simulink model "mrefrobotarm_previous_y_previous_u_previous_ref_cover_test_2"  (R2018b)
settings: Solver=FixedStepAuto  StartTime=0.0  StopTime=20  RelTol=1e-3  AbsTol=1e-6
undefined symbols (not defined in the file or in its folder): cc, options
libraries: neural x132, simulink x2
(part 4 of 6)

== system mrefrobotarm_previous_y_previous_u_previous_ref_cover_test_2/Feed-Forward Neural Network/Layer 3/Delays 1 ==
  "p{3}" : Inport  PortDimensions=30
      mask Display: e = 0.06;c1 = [120 230 180]/255;c2 = ([120 230 180]+0)/(256+128);c3 = ([120 230 180]+128)/(256+128);patch([0 1 1 0],[0 0 1 1],c1);patch([0 1 1 1-e 1-e 0+e],[0 0 1 1-e 0+e 0+e],c2);patch([0 0 1 1-e 0+e 0+e],[0 1 1 1-e 1-e 0+e],c3);plot([0 1 1 0 0],[0 0 1 1 0]);
  mux : Mux  Inputs=1
      mask Display: e = 0.06;c1 = [120 150 230]/255;c2 = ([120 150 230]+0)/383;c3 = ([120 150 230]+128)/383;patch([0 1 1 0],[0 0 1 1],c1);patch([0 1 1 1-e 1-e 0+e],[0 0 1 1-e 0+e 0+e],c2);patch([0 0 1 1-e 0+e 0+e],[0 1 1 1-e 1-e 0+e],c3);plot([0 1 1 0 0],[0 0 1 1 0]);disp('Mux')
  "pd{3,2}" : Outport
      mask Display: e = 0.06;c1 = [120 230 180]/255;c2 = ([120 230 180]+0)/(256+128);c3 = ([120 230 180]+128)/(256+128);patch([0 1 1 0],[0 0 1 1],c1);patch([0 1 1 1-e 1-e 0+e],[0 0 1 1-e 0+e 0+e],c2);patch([0 0 1 1-e 0+e 0+e],[0 1 1 1-e 1-e 0+e],c3);plot([0 1 1 0 0],[0 0 1 1 0]);
  wires:
  "p{3}"/1 -> mux/1
  mux/1 -> "pd{3,2}"/1

== system mrefrobotarm_previous_y_previous_u_previous_ref_cover_test_2/Feed-Forward Neural Network/Layer 3/LW{3,2} ==
  "ad{3,2}" : Inport  PortDimensions=30
      mask Display: e = 0.06;c1 = [120 230 180]/255;c2 = ([120 230 180]+0)/(256+128);c3 = ([120 230 180]+128)/(256+128);patch([0 1 1 0],[0 0 1 1],c1);patch([0 1 1 1-e 1-e 0+e],[0 0 1 1-e 0+e 0+e],c2);patch([0 0 1 1-e 0+e 0+e],[0 1 1 1-e 1-e 0+e],c3);plot([0 1 1 0 0],[0 0 1 1 0]);
  "IW{3,2}(1,:)'" : Constant  Value=[-0.179633159964680266806880126750911585986614227294921875;-0.01072873765062364037614628387018456123769283294677734375;-0.0291453057248748058360998669513719505630433559417724609375;0.05859045612955075810202032471352140419185161590576171875;-0.237638764700321913903025006220559589564800262451171875;-0.209838527725091539277713081901310943067073822021484375;-0.27791655307496510030063063823035918176174163818359375;-0.07008976059233355815347721318175899796187877655029296875;-0.11554327471293225626514100667918683029711246490478515625;0.27212249906517038677833397741778753697872161865234375;-0.1734031338030869451305449047140427865087985992431640625;0.0536763624525791460673218580268439836800098419189453125;-0.037173437880853761605681739865758572705090045928955078125;0.1358518131119930971717479906146763823926448822021484375;-0.11157815841815578450368917629020870663225650787353515625;-0.023913464068717076027592582931902143172919750213623046875;-0.4313994517536372530486232790281064808368682861328125;0.1636875861604869808463291747102630324661731719970703125;0.037232113811342650022684352961732656694948673248291015625;-0.52644415726454052428806562602403573691844940185546875;0.039897217969779720514456045066253864206373691558837890625;-0.1369287872106144388073545314910006709396839141845703125;0.44593864887069745162051503939437679946422576904296875;0.410742338437982856813590615274733863770961761474609375;-0.145121658875231818175421949490555562078952789306640625;0.06655502995710448066457587401600903831422328948974609375;-0.418109406113754300537976860141498036682605743408203125;0.11096998879556761730125202802810235880315303802490234375;0.333827163986122277261614499366260133683681488037109375;0.186101897373585012385177606120123527944087982177734375]
      mask Display: e = 0.06;c1 = [120 150 230]/255;c2 = ([120 150 230]+0)/383;c3 = ([120 150 230]+128)/383;patch([0 1 1 0],[0 0 1 1],c1);patch([0 1 1 1-e 1-e 0+e],[0 0 1 1-e 0+e 0+e],c2);patch([0 0 1 1-e 0+e 0+e],[0 1 1 1-e 1-e 0+e],c3);plot([0 1 1 0 0],[0 0 1 1 0]);disp('weights');
  Mux : Mux  Inputs=1
      mask Display: e = 0.06;c1 = [120 150 230]/255;c2 = ([120 150 230]+0)/383;c3 = ([120 150 230]+128)/383;patch([0 1 1 0],[0 0 1 1],c1);patch([0 1 1 1-e 1-e 0+e],[0 0 1 1-e 0+e 0+e],c2);patch([0 0 1 1-e 0+e 0+e],[0 1 1 1-e 1-e 0+e],c3);plot([0 1 1 0 0],[0 0 1 1 0]);disp('Mux');
  dotprod1 : neural/Weight Functions/dotprod
  "lz{3,2}" : Outport
      mask Display: e = 0.06;c1 = [120 230 180]/255;c2 = ([120 230 180]+0)/(256+128);c3 = ([120 230 180]+128)/(256+128);patch([0 1 1 0],[0 0 1 1],c1);patch([0 1 1 1-e 1-e 0+e],[0 0 1 1-e 0+e 0+e],c2);patch([0 0 1 1-e 0+e 0+e],[0 1 1 1-e 1-e 0+e],c3);plot([0 1 1 0 0],[0 0 1 1 0]);
  wires:
  "IW{3,2}(1,:)'"/1 -> dotprod1/1
  "ad{3,2}"/1 -> dotprod1/2
  dotprod1/1 -> Mux/1
  Mux/1 -> "lz{3,2}"/1

== system mrefrobotarm_previous_y_previous_u_previous_ref_cover_test_2/Feed-Forward Neural Network1/Layer 1/Delays 1 ==
  "p{1}" : Inport  PortDimensions=10
      mask Display: e = 0.06;c1 = [120 230 180]/255;c2 = ([120 230 180]+0)/(256+128);c3 = ([120 230 180]+128)/(256+128);patch([0 1 1 0],[0 0 1 1],c1);patch([0 1 1 1-e 1-e 0+e],[0 0 1 1-e 0+e 0+e],c2);patch([0 0 1 1-e 0+e 0+e],[0 1 1 1-e 1-e 0+e],c3);plot([0 1 1 0 0],[0 0 1 1 0]);
  mux : Mux  Inputs=1
      mask Display: e = 0.06;c1 = [120 150 230]/255;c2 = ([120 150 230]+0)/383;c3 = ([120 150 230]+128)/383;patch([0 1 1 0],[0 0 1 1],c1);patch([0 1 1 1-e 1-e 0+e],[0 0 1 1-e 0+e 0+e],c2);patch([0 0 1 1-e 0+e 0+e],[0 1 1 1-e 1-e 0+e],c3);plot([0 1 1 0 0],[0 0 1 1 0]);disp('Mux')
  "pd{1,1}" : Outport
      mask Display: e = 0.06;c1 = [120 230 180]/255;c2 = ([120 230 180]+0)/(256+128);c3 = ([120 230 180]+128)/(256+128);patch([0 1 1 0],[0 0 1 1],c1);patch([0 1 1 1-e 1-e 0+e],[0 0 1 1-e 0+e 0+e],c2);patch([0 0 1 1-e 0+e 0+e],[0 1 1 1-e 1-e 0+e],c3);plot([0 1 1 0 0],[0 0 1 1 0]);
  wires:
  "p{1}"/1 -> mux/1
  mux/1 -> "pd{1,1}"/1

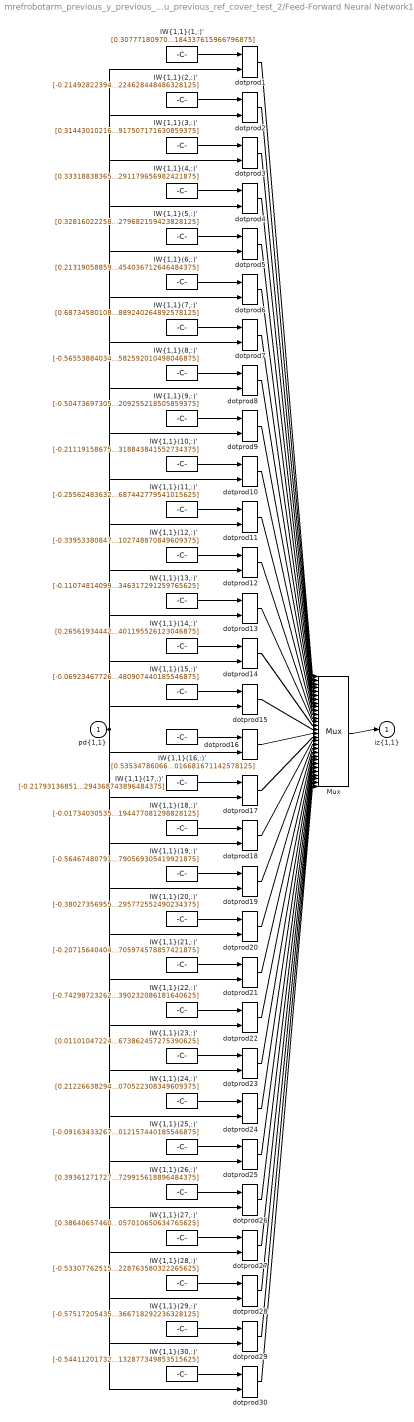
== system mrefrobotarm_previous_y_previous_u_previous_ref_cover_test_2/Feed-Forward Neural Network1/Layer 1/IW{1,1} ==
  "pd{1,1}" : Inport  PortDimensions=10
      mask Display: e = 0.06;c1 = [120 230 180]/255;c2 = ([120 230 180]+0)/(256+128);c3 = ([120 230 180]+128)/(256+128);patch([0 1 1 0],[0 0 1 1],c1);patch([0 1 1 1-e 1-e 0+e],[0 0 1 1-e 0+e 0+e],c2);patch([0 0 1 1-e 0+e 0+e],[0 1 1 1-e 1-e 0+e],c3);plot([0 1 1 0 0],[0 0 1 1 0]);
  "IW{1,1}(1,:)'" : Constant  Value=[0.307771809704280141506416157426428981125354766845703125;-0.043494246471554913469059755470880190841853618621826171875;-0.038310852488129772119851423894942854531109333038330078125;-0.39541211499447570520970884899725206196308135986328125;-0.70069751174348116062873259579646401107311248779296875;0.65787882665114827407393249814049340784549713134765625;-0.444848337035453955667918535255012102425098419189453125;-0.534193590442934240769545795046724379062652587890625;-0.452507108681440561870346073192195035517215728759765625;0.5736423354881441394326202498632483184337615966796875]
      mask Display: e = 0.06;c1 = [120 150 230]/255;c2 = ([120 150 230]+0)/383;c3 = ([120 150 230]+128)/383;patch([0 1 1 0],[0 0 1 1],c1);patch([0 1 1 1-e 1-e 0+e],[0 0 1 1-e 0+e 0+e],c2);patch([0 0 1 1-e 0+e 0+e],[0 1 1 1-e 1-e 0+e],c3);plot([0 1 1 0 0],[0 0 1 1 0]);disp('Weights');
  "IW{1,1}(10,:)'" : Constant  Value=[-0.2111915867591773465772320150790619663894176483154296875;-0.42392787982224933163166724625625647604465484619140625;0.313182134356018437859603409378905780613422393798828125;0.8660538287659613754243537186994217336177825927734375;0.465944929849588296288942501632845960557460784912109375;-0.317882144322859605534148386141168884932994842529296875;0.5471005603664356176096816852805204689502716064453125;0.048378896684587037457792035866077640093863010406494140625;0.88527457170474466163767601756262592971324920654296875;-0.06293203749796126567073173418975784443318843841552734375]
      mask Display: e = 0.06;c1 = [120 150 230]/255;c2 = ([120 150 230]+0)/383;c3 = ([120 150 230]+128)/383;patch([0 1 1 0],[0 0 1 1],c1);patch([0 1 1 1-e 1-e 0+e],[0 0 1 1-e 0+e 0+e],c2);patch([0 0 1 1-e 0+e 0+e],[0 1 1 1-e 1-e 0+e],c3);plot([0 1 1 0 0],[0 0 1 1 0]);disp('Weights');
  "IW{1,1}(11,:)'" : Constant  Value=[-0.255624836328040394572980176235432736575603485107421875;0.44469153543896167146698417127481661736965179443359375;0.58810225130934201676069505992927588522434234619140625;-0.381773211793491717980231214824016205966472625732421875;0.636150888388204549528381903655827045440673828125;-0.160165825236976699930124823367805220186710357666015625;0.361341451607977981463903915937407873570919036865234375;0.428811830416127082177268903251388110220432281494140625;-0.372886982074612571835814378573559224605560302734375;0.401883345447998918675835966496379114687442779541015625]
      mask Display: e = 0.06;c1 = [120 150 230]/255;c2 = ([120 150 230]+0)/383;c3 = ([120 150 230]+128)/383;patch([0 1 1 0],[0 0 1 1],c1);patch([0 1 1 1-e 1-e 0+e],[0 0 1 1-e 0+e 0+e],c2);patch([0 0 1 1-e 0+e 0+e],[0 1 1 1-e 1-e 0+e],c3);plot([0 1 1 0 0],[0 0 1 1 0]);disp('Weights');
  "IW{1,1}(12,:)'" : Constant  Value=[-0.339533808477128939973255228323978371918201446533203125;0.539710960120284966023973538540303707122802734375;-0.7230875453157439292084518456249497830867767333984375;-0.75990866812186597112344088600366376340389251708984375;-0.354088287837987625294999816105701029300689697265625;-0.353970240989271711651298346623661927878856658935546875;-0.10842578628777639615510253179309074766933917999267578125;-0.01447441056256725845641231131821768940426409244537353515625;-0.456615513925438809561541120274341665208339691162109375;-0.261220551168401760033788150394684635102748870849609375]
      mask Display: e = 0.06;c1 = [120 150 230]/255;c2 = ([120 150 230]+0)/383;c3 = ([120 150 230]+128)/383;patch([0 1 1 0],[0 0 1 1],c1);patch([0 1 1 1-e 1-e 0+e],[0 0 1 1-e 0+e 0+e],c2);patch([0 0 1 1-e 0+e 0+e],[0 1 1 1-e 1-e 0+e],c3);plot([0 1 1 0 0],[0 0 1 1 0]);disp('Weights');
  "IW{1,1}(13,:)'" : Constant  Value=[-0.110748140990551302564881552825681865215301513671875;0.66488624107314231448384589384659193456172943115234375;-1.00451912367756523991602080059237778186798095703125;-0.0143360503455160250008137978738886886276304721832275390625;0.6747034829726137328265167525387369096279144287109375;0.037869992030076689293327518726073321886360645294189453125;-0.2233703071642894055770511840819381177425384521484375;0.1543495324337380847357081847803783603012561798095703125;-0.6817280066758144574379230107297189533710479736328125;-0.25424477166286740814626909923390485346317291259765625]
      mask Display: e = 0.06;c1 = [120 150 230]/255;c2 = ([120 150 230]+0)/383;c3 = ([120 150 230]+128)/383;patch([0 1 1 0],[0 0 1 1],c1);patch([0 1 1 1-e 1-e 0+e],[0 0 1 1-e 0+e 0+e],c2);patch([0 0 1 1-e 0+e 0+e],[0 1 1 1-e 1-e 0+e],c3);plot([0 1 1 0 0],[0 0 1 1 0]);disp('Weights');
  "IW{1,1}(14,:)'" : Constant  Value=[0.265619344429818438069190733585855923593044281005859375;-0.282970550854229341286583121473086066544055938720703125;-0.5838578775873510817717715326580218970775604248046875;0.294580978398594428568912917398847639560699462890625;0.64224270360970781013065789011307060718536376953125;-0.17698999119896263731988028666819445788860321044921875;-0.06350503851383948461517547912080772221088409423828125;0.58935462278309425077083005817257799208164215087890625;0.62621659979370136728249462976236827671527862548828125;0.1318430666219640723380024383004638366401195526123046875]
      mask Display: e = 0.06;c1 = [120 150 230]/255;c2 = ([120 150 230]+0)/383;c3 = ([120 150 230]+128)/383;patch([0 1 1 0],[0 0 1 1],c1);patch([0 1 1 1-e 1-e 0+e],[0 0 1 1-e 0+e 0+e],c2);patch([0 0 1 1-e 0+e 0+e],[0 1 1 1-e 1-e 0+e],c3);plot([0 1 1 0 0],[0 0 1 1 0]);disp('Weights');
  "IW{1,1}(15,:)'" : Constant  Value=[-0.069234677267842936743136306176893413066864013671875;0.357620645651575530532539914929657243192195892333984375;0.024739682030093586295738106173303094692528247833251953125;0.406580565759079914922580201164237223565578460693359375;-0.1414763552845024197068823923473246395587921142578125;0.77379347285040334103456416414701379835605621337890625;0.54400482337093336582256597466766834259033203125;0.257672646340499966743919912914861924946308135986328125;0.4042055275314468953951063667773269116878509521484375;0.6191001141682999087123562276246957480907440185546875]
      mask Display: e = 0.06;c1 = [120 150 230]/255;c2 = ([120 150 230]+0)/383;c3 = ([120 150 230]+128)/383;patch([0 1 1 0],[0 0 1 1],c1);patch([0 1 1 1-e 1-e 0+e],[0 0 1 1-e 0+e 0+e],c2);patch([0 0 1 1-e 0+e 0+e],[0 1 1 1-e 1-e 0+e],c3);plot([0 1 1 0 0],[0 0 1 1 0]);disp('Weights');
  "IW{1,1}(16,:)'" : Constant  Value=[0.5353478606635488912246501058689318597316741943359375;-0.298798871045879599339656351730809547007083892822265625;-0.306842919989221252219380176029517315328121185302734375;0.79214491503970763108810615449328906834125518798828125;0.107274974298643910319839278599829412996768951416015625;-0.04982289745277827808234150097632664255797863006591796875;0.1398078294476846339389197737546055577695369720458984375;0.73950277251963658642353038885630667209625244140625;0.0214329040625382515050656451194299734197556972503662109375;-0.59363821103110503418776033868198283016681671142578125]
      mask Display: e = 0.06;c1 = [120 150 230]/255;c2 = ([120 150 230]+0)/383;c3 = ([120 150 230]+128)/383;patch([0 1 1 0],[0 0 1 1],c1);patch([0 1 1 1-e 1-e 0+e],[0 0 1 1-e 0+e 0+e],c2);patch([0 0 1 1-e 0+e 0+e],[0 1 1 1-e 1-e 0+e],c3);plot([0 1 1 0 0],[0 0 1 1 0]);disp('Weights');
  "IW{1,1}(17,:)'" : Constant  Value=[-0.2179313685150011392632762863286188803613185882568359375;0.02389454008851725486106687412757310084998607635498046875;0.80226571345702046844650112689123488962650299072265625;0.33127862043797751123719308452564291656017303466796875;-0.47181821059433415310735426828614436089992523193359375;0.0302617469843945753604774751011063926853239536285400390625;0.78373483792398135339141163058229722082614898681640625;-0.033101967548309345346080334593352745287120342254638671875;-0.06509617185323690602416490946779958903789520263671875;-0.4540540617562258685069309649406932294368743896484375]
      mask Display: e = 0.06;c1 = [120 150 230]/255;c2 = ([120 150 230]+0)/383;c3 = ([120 150 230]+128)/383;patch([0 1 1 0],[0 0 1 1],c1);patch([0 1 1 1-e 1-e 0+e],[0 0 1 1-e 0+e 0+e],c2);patch([0 0 1 1-e 0+e 0+e],[0 1 1 1-e 1-e 0+e],c3);plot([0 1 1 0 0],[0 0 1 1 0]);disp('Weights');
  "IW{1,1}(18,:)'" : Constant  Value=[-0.017340305353522177111980084873721352778375148773193359375;0.04635262968849508669055836662664660252630710601806640625;0.49087893166783247433926362646161578595638275146484375;0.261355444844639184243106910798815079033374786376953125;0.038895872356487219689835654889975558035075664520263671875;0.76061985589617275849150246358476579189300537109375;0.16038243618602454620969410825637169182300567626953125;0.269770227677864460336110141724930144846439361572265625;0.85486484585484101561547731762402690947055816650390625;-0.474622970419836420763459727822919376194477081298828125]
      mask Display: e = 0.06;c1 = [120 150 230]/255;c2 = ([120 150 230]+0)/383;c3 = ([120 150 230]+128)/383;patch([0 1 1 0],[0 0 1 1],c1);patch([0 1 1 1-e 1-e 0+e],[0 0 1 1-e 0+e 0+e],c2);patch([0 0 1 1-e 0+e 0+e],[0 1 1 1-e 1-e 0+e],c3);plot([0 1 1 0 0],[0 0 1 1 0]);disp('Weights');
  "IW{1,1}(19,:)'" : Constant  Value=[-0.56467480791342705703783622084301896393299102783203125;-0.0030660566154840085406618754859664477407932281494140625;-0.342498503655595476491413364783511497080326080322265625;-0.22528161666232360271777679372462444007396697998046875;0.06229949556277590561048640438457368873059749603271484375;-0.856195965195246433410147801623679697513580322265625;0.56695735295288007815628361640847288072109222412109375;-0.18273876771567143517671638619503937661647796630859375;-0.39019604298290000432558599641197361052036285400390625;-0.643270272670612097698494835640303790569305419921875]
      mask Display: e = 0.06;c1 = [120 150 230]/255;c2 = ([120 150 230]+0)/383;c3 = ([120 150 230]+128)/383;patch([0 1 1 0],[0 0 1 1],c1);patch([0 1 1 1-e 1-e 0+e],[0 0 1 1-e 0+e 0+e],c2);patch([0 0 1 1-e 0+e 0+e],[0 1 1 1-e 1-e 0+e],c3);plot([0 1 1 0 0],[0 0 1 1 0]);disp('Weights');
  "IW{1,1}(2,:)'" : Constant  Value=[-0.2149282239453440268572848026451538316905498504638671875;0.50939800546889235643988058654940687119960784912109375;-0.570595278838305741686554029001854360103607177734375;-0.6491838212484617454123281277134083211421966552734375;0.524588753903739490880298035335727035999298095703125;-0.325806575234383277717142846086062490940093994140625;0.4073454672740408621933738686493597924709320068359375;0.1445179480051441978094572959889774210751056671142578125;0.557599898389703252377103126491419970989227294921875;-0.33629203092728687796153508315910585224628448486328125]
      mask Display: e = 0.06;c1 = [120 150 230]/255;c2 = ([120 150 230]+0)/383;c3 = ([120 150 230]+128)/383;patch([0 1 1 0],[0 0 1 1],c1);patch([0 1 1 1-e 1-e 0+e],[0 0 1 1-e 0+e 0+e],c2);patch([0 0 1 1-e 0+e 0+e],[0 1 1 1-e 1-e 0+e],c3);plot([0 1 1 0 0],[0 0 1 1 0]);disp('Weights');
  "IW{1,1}(20,:)'" : Constant  Value=[-0.380273569552752876976597917746403254568576812744140625;-0.430511165009204999076786180012277327477931976318359375;0.354253288781558206554933576626353897154331207275390625;0.445619148653988272901216305399429984390735626220703125;-0.60980214170925106653697866931906901299953460693359375;0.60264849482189231100193183010560460388660430908203125;0.286226129170386867084374671321711502969264984130859375;0.296664076206746951669401823892258107662200927734375;-0.38376606122486578431818315948476083576679229736328125;0.1592426923493431567546707583460374735295772552490234375]
      mask Display: e = 0.06;c1 = [120 150 230]/255;c2 = ([120 150 230]+0)/383;c3 = ([120 150 230]+128)/383;patch([0 1 1 0],[0 0 1 1],c1);patch([0 1 1 1-e 1-e 0+e],[0 0 1 1-e 0+e 0+e],c2);patch([0 0 1 1-e 0+e 0+e],[0 1 1 1-e 1-e 0+e],c3);plot([0 1 1 0 0],[0 0 1 1 0]);disp('Weights');
  "IW{1,1}(21,:)'" : Constant  Value=[-0.20715640404519952699757823211257345974445343017578125;0.9811699028163343161423881610971875488758087158203125;-0.001095329187504811944975369186749958316795527935028076171875;-0.277444713932339770412482948813703842461109161376953125;0.55580805253002185661870271360385231673717498779296875;-0.64553407503771043085549763418384827673435211181640625;-0.422001384311685712180661766979028470814228057861328125;0.393923183878474636454569690613425336778163909912109375;0.083918194813454027869425999597297050058841705322265625;-0.283713183453508654974228875289554707705974578857421875]
      mask Display: e = 0.06;c1 = [120 150 230]/255;c2 = ([120 150 230]+0)/383;c3 = ([120 150 230]+128)/383;patch([0 1 1 0],[0 0 1 1],c1);patch([0 1 1 1-e 1-e 0+e],[0 0 1 1-e 0+e 0+e],c2);patch([0 0 1 1-e 0+e 0+e],[0 1 1 1-e 1-e 0+e],c3);plot([0 1 1 0 0],[0 0 1 1 0]);disp('Weights');
  "IW{1,1}(22,:)'" : Constant  Value=[-0.74298723262986421378428758544032461941242218017578125;-0.474285430413762976176172969644539989531040191650390625;-0.2219220129482323555780709511964232660830020904541015625;-0.07774456600170388809178945166422636248171329498291015625;0.159011878942632634004183955767075531184673309326171875;-0.474236493815869242229865676563349552452564239501953125;-0.34955980920388896038275561295449733734130859375;0.263576614616158944048862622366868890821933746337890625;0.656227952555379356880393970641307532787322998046875;0.495996797371051345582060321248718537390232086181640625]
      mask Display: e = 0.06;c1 = [120 150 230]/255;c2 = ([120 150 230]+0)/383;c3 = ([120 150 230]+128)/383;patch([0 1 1 0],[0 0 1 1],c1);patch([0 1 1 1-e 1-e 0+e],[0 0 1 1-e 0+e 0+e],c2);patch([0 0 1 1-e 0+e 0+e],[0 1 1 1-e 1-e 0+e],c3);plot([0 1 1 0 0],[0 0 1 1 0]);disp('Weights');
  "IW{1,1}(23,:)'" : Constant  Value=[0.01101047224694271138567547296815973822958767414093017578125;-0.83652318268884062746337804128415882587432861328125;-0.6720858263646014574277387509937398135662078857421875;0.06519613312673551430709295573251438327133655548095703125;-0.288183944151695625723874627510667778551578521728515625;-0.48909683596764808033441340739955194294452667236328125;0.54268768030462333218366666187648661434650421142578125;-0.0153055303761240289739387065992559655569493770599365234375;0.1757264020219303224390472450977540574967861175537109375;-0.293937485561877986928180916947894729673862457275390625]
      mask Display: e = 0.06;c1 = [120 150 230]/255;c2 = ([120 150 230]+0)/383;c3 = ([120 150 230]+128)/383;patch([0 1 1 0],[0 0 1 1],c1);patch([0 1 1 1-e 1-e 0+e],[0 0 1 1-e 0+e 0+e],c2);patch([0 0 1 1-e 0+e 0+e],[0 1 1 1-e 1-e 0+e],c3);plot([0 1 1 0 0],[0 0 1 1 0]);disp('Weights');
  "IW{1,1}(24,:)'" : Constant  Value=[0.2122663829425259496286315652469056658446788787841796875;0.87923061827891757502584368921816349029541015625;-0.5173249006417501849597329055541194975376129150390625;-0.50307150349048967985510216749389655888080596923828125;0.1947665745272291193401770215132273733615875244140625;0.26726591958569378970622665292466990649700164794921875;-0.128537570280304602743370878670248202979564666748046875;-0.4015021175823199062193680219934321939945220947265625;0.71182418664467472790846613861504010856151580810546875;-0.122855789206089749399097854620777070522308349609375]
      mask Display: e = 0.06;c1 = [120 150 230]/255;c2 = ([120 150 230]+0)/383;c3 = ([120 150 230]+128)/383;patch([0 1 1 0],[0 0 1 1],c1);patch([0 1 1 1-e 1-e 0+e],[0 0 1 1-e 0+e 0+e],c2);patch([0 0 1 1-e 0+e 0+e],[0 1 1 1-e 1-e 0+e],c3);plot([0 1 1 0 0],[0 0 1 1 0]);disp('Weights');
  "IW{1,1}(25,:)'" : Constant  Value=[-0.09163433267084818145686853085862821899354457855224609375;-0.79242044992990423590839554890408180654048919677734375;-0.100048388071002858357161358071607537567615509033203125;0.1508863568801963317422831778458203189074993133544921875;-0.52491946330139238607870311170700006186962127685546875;-0.9073207461986847466306471687857992947101593017578125;0.305921576666395356181027409547823481261730194091796875;-0.28550897310796197192672707387828268110752105712890625;0.3700650003189187575713958722190000116825103759765625;0.01483537959348367289702519400407254579477012157440185546875]
      mask Display: e = 0.06;c1 = [120 150 230]/255;c2 = ([120 150 230]+0)/383;c3 = ([120 150 230]+128)/383;patch([0 1 1 0],[0 0 1 1],c1);patch([0 1 1 1-e 1-e 0+e],[0 0 1 1-e 0+e 0+e],c2);patch([0 0 1 1-e 0+e 0+e],[0 1 1 1-e 1-e 0+e],c3);plot([0 1 1 0 0],[0 0 1 1 0]);disp('Weights');
  "IW{1,1}(26,:)'" : Constant  Value=[0.393612717278230495043800374332931824028491973876953125;0.2449765807941226558597236362402327358722686767578125;-0.03009018765526084993044975135489949025213718414306640625;0.14629061622603833914268989246920682489871978759765625;0.439887108136198412555728509687469340860843658447265625;0.435562173454939915995254295921768061816692352294921875;0.336788968183238723863581753903417848050594329833984375;-0.428207393410589443050184854655526578426361083984375;-0.054417900950539950521989140952427987940609455108642578125;1.0199853001420409182031789896427653729915618896484375]
      mask Display: e = 0.06;c1 = [120 150 230]/255;c2 = ([120 150 230]+0)/383;c3 = ([120 150 230]+128)/383;patch([0 1 1 0],[0 0 1 1],c1);patch([0 1 1 1-e 1-e 0+e],[0 0 1 1-e 0+e 0+e],c2);patch([0 0 1 1-e 0+e 0+e],[0 1 1 1-e 1-e 0+e],c3);plot([0 1 1 0 0],[0 0 1 1 0]);disp('Weights');
  "IW{1,1}(27,:)'" : Constant  Value=[0.386406574607860431314065863261930644512176513671875;0.469835350060989143106127130522509105503559112548828125;-0.3691521633424239556831025765859521925449371337890625;-0.45968636278126029370838523391284979879856109619140625;-0.12253896032814211303207940773063455708324909210205078125;0.51055111602274383386657063965685665607452392578125;-0.25427556952147067903524657594971358776092529296875;0.4000694399878466089859330168110318481922149658203125;0.5497090132858077904387528178631328046321868896484375;0.62451276436301006445006578360334970057010650634765625]
      mask Display: e = 0.06;c1 = [120 150 230]/255;c2 = ([120 150 230]+0)/383;c3 = ([120 150 230]+128)/383;patch([0 1 1 0],[0 0 1 1],c1);patch([0 1 1 1-e 1-e 0+e],[0 0 1 1-e 0+e 0+e],c2);patch([0 0 1 1-e 0+e 0+e],[0 1 1 1-e 1-e 0+e],c3);plot([0 1 1 0 0],[0 0 1 1 0]);disp('Weights');
  "IW{1,1}(28,:)'" : Constant  Value=[-0.5330776251530677800616331296623684465885162353515625;-0.09896275413630002681930619701233808882534503936767578125;0.59870269426114497424151750237797386944293975830078125;0.6583543298551373101901162954163737595081329345703125;0.62137262912390955893471300441888161003589630126953125;0.0274271679633210745119509255118828150443732738494873046875;-0.386383313608881895362401337479241192340850830078125;-0.373521518345400205252104797182255424559116363525390625;-0.1745289113787924784038096959193353541195392608642578125;-0.68166057721812711722719768658862449228763580322265625]
      mask Display: e = 0.06;c1 = [120 150 230]/255;c2 = ([120 150 230]+0)/383;c3 = ([120 150 230]+128)/383;patch([0 1 1 0],[0 0 1 1],c1);patch([0 1 1 1-e 1-e 0+e],[0 0 1 1-e 0+e 0+e],c2);patch([0 0 1 1-e 0+e 0+e],[0 1 1 1-e 1-e 0+e],c3);plot([0 1 1 0 0],[0 0 1 1 0]);disp('Weights');
  "IW{1,1}(29,:)'" : Constant  Value=[-0.57517205435042340067042232476524077355861663818359375;0.63308192763810922087941435165703296661376953125;-0.09556525966967858998213358745488221757113933563232421875;-0.5584199775632636697508814904722385108470916748046875;0.345765858847536577957981762665440328419208526611328125;0.08596895869872944739853437567944638431072235107421875;-0.1846575835968873591230732245094259269535541534423828125;0.65145079957593632347112588831805624067783355712890625;-0.501689780634055892960532219149172306060791015625;-0.61266191132330505286773814077605493366718292236328125]
      mask Display: e = 0.06;c1 = [120 150 230]/255;c2 = ([120 150 230]+0)/383;c3 = ([120 150 230]+128)/383;patch([0 1 1 0],[0 0 1 1],c1);patch([0 1 1 1-e 1-e 0+e],[0 0 1 1-e 0+e 0+e],c2);patch([0 0 1 1-e 0+e 0+e],[0 1 1 1-e 1-e 0+e],c3);plot([0 1 1 0 0],[0 0 1 1 0]);disp('Weights');
  "IW{1,1}(3,:)'" : Constant  Value=[0.314430102162298330537026913589215837419033050537109375;0.276695513253253644325724280861322768032550811767578125;0.11751958538400335274598518253696965985000133514404296875;0.1846764705887174173870590720980544574558734893798828125;-0.64765345192008594299437618246884085237979888916015625;-0.69717973432415181189725217336672358214855194091796875;0.1215129375684755042019702386824064888060092926025390625;0.38445320860246934291382103765499778091907501220703125;0.74698130652669891826889170260983519256114959716796875;0.297597636979915092236836926531395874917507171630859375]
      mask Display: e = 0.06;c1 = [120 150 230]/255;c2 = ([120 150 230]+0)/383;c3 = ([120 150 230]+128)/383;patch([0 1 1 0],[0 0 1 1],c1);patch([0 1 1 1-e 1-e 0+e],[0 0 1 1-e 0+e 0+e],c2);patch([0 0 1 1-e 0+e 0+e],[0 1 1 1-e 1-e 0+e],c3);plot([0 1 1 0 0],[0 0 1 1 0]);disp('Weights');
  "IW{1,1}(30,:)'" : Constant  Value=[-0.54411201732523573060262833678280003368854522705078125;-0.1570049627788529245098203546149306930601596832275390625;0.4750648553590675060576131727430038154125213623046875;-0.332924171479602348799886613051057793200016021728515625;0.336816257924666573320138240887899883091449737548828125;0.0772141881037635702256238801055587828159332275390625;0.138879371464563750038223588489927351474761962890625;-0.7413902499064313200705100825871340930461883544921875;-0.556925916111620011861305101774632930755615234375;-0.379493537000827940719460684704245068132877349853515625]
      mask Display: e = 0.06;c1 = [120 150 230]/255;c2 = ([120 150 230]+0)/383;c3 = ([120 150 230]+128)/383;patch([0 1 1 0],[0 0 1 1],c1);patch([0 1 1 1-e 1-e 0+e],[0 0 1 1-e 0+e 0+e],c2);patch([0 0 1 1-e 0+e 0+e],[0 1 1 1-e 1-e 0+e],c3);plot([0 1 1 0 0],[0 0 1 1 0]);disp('Weights');
  "IW{1,1}(4,:)'" : Constant  Value=[0.333188383657982922780860235434374772012233734130859375;-0.8119891062851021246160598821006715297698974609375;-0.43539581511156633109038693874026648700237274169921875;0.115329974937103341137145662287366576492786407470703125;-0.410897767185643358889279852519393898546695709228515625;-0.1653380888177397867178086698913830332458019256591796875;-0.66921948665613950613106908349436707794666290283203125;0.2423332585656756965608593645811197347939014434814453125;0.352153723637267657142757570909452624619007110595703125;-0.471892129319398001552343657749588601291179656982421875]
      mask Display: e = 0.06;c1 = [120 150 230]/255;c2 = ([120 150 230]+0)/383;c3 = ([120 150 230]+128)/383;patch([0 1 1 0],[0 0 1 1],c1);patch([0 1 1 1-e 1-e 0+e],[0 0 1 1-e 0+e 0+e],c2);patch([0 0 1 1-e 0+e 0+e],[0 1 1 1-e 1-e 0+e],c3);plot([0 1 1 0 0],[0 0 1 1 0]);disp('Weights');
  "IW{1,1}(5,:)'" : Constant  Value=[0.328160222582545901826023282410460524260997772216796875;0.11696869091104332427644152403445332311093807220458984375;-0.56572687517270459078844169198418967425823211669921875;-0.044997049681217267391719616398404468782246112823486328125;-0.414037671684482855294362479980918578803539276123046875;-0.6718978551824748013387988976319320499897003173828125;0.11602708978398555694777627422809018753468990325927734375;-0.28088853726513984820911673523369245231151580810546875;-0.1101044169173044096066149677426437847316265106201171875;0.72922980289897498806794828851707279682159423828125]
      mask Display: e = 0.06;c1 = [120 150 230]/255;c2 = ([120 150 230]+0)/383;c3 = ([120 150 230]+128)/383;patch([0 1 1 0],[0 0 1 1],c1);patch([0 1 1 1-e 1-e 0+e],[0 0 1 1-e 0+e 0+e],c2);patch([0 0 1 1-e 0+e 0+e],[0 1 1 1-e 1-e 0+e],c3);plot([0 1 1 0 0],[0 0 1 1 0]);disp('Weights');
  "IW{1,1}(6,:)'" : Constant  Value=[0.2131905885959748669922220187800121493637561798095703125;-0.5860198782401695449806311444262973964214324951171875;-0.025722683958631163692043486435068189166486263275146484375;-0.423381128821053220878667389115435071289539337158203125;-0.5299260658931281842143334870343096554279327392578125;-0.2127867716926119812104190032187034375965595245361328125;-0.82213091748145739057207492805900983512401580810546875;0.128184993846583827892260387670830823481082916259765625;-0.403831106100383807611109432400553487241268157958984375;-0.294851875606935764917437836629687808454036712646484375]
      mask Display: e = 0.06;c1 = [120 150 230]/255;c2 = ([120 150 230]+0)/383;c3 = ([120 150 230]+128)/383;patch([0 1 1 0],[0 0 1 1],c1);patch([0 1 1 1-e 1-e 0+e],[0 0 1 1-e 0+e 0+e],c2);patch([0 0 1 1-e 0+e 0+e],[0 1 1 1-e 1-e 0+e],c3);plot([0 1 1 0 0],[0 0 1 1 0]);disp('Weights');
  "IW{1,1}(7,:)'" : Constant  Value=[0.68734580108934728581715489781345240771770477294921875;-0.281842547917039165650265886142733506858348846435546875;-0.416611576017458740128773797550820745527744293212890625;0.08339783305877103425363117139568203128874301910400390625;0.6320326138479421818061609883443452417850494384765625;-0.045489126505797179700341104080507648177444934844970703125;-0.0185403344429965373507673831454667379148304462432861328125;-0.45736662772395375586853560889721848070621490478515625;0.82203309649191813601731837479746900498867034912109375;0.459313596929332768059595082377200014889240264892578125]
      mask Display: e = 0.06;c1 = [120 150 230]/255;c2 = ([120 150 230]+0)/383;c3 = ([120 150 230]+128)/383;patch([0 1 1 0],[0 0 1 1],c1);patch([0 1 1 1-e 1-e 0+e],[0 0 1 1-e 0+e 0+e],c2);patch([0 0 1 1-e 0+e 0+e],[0 1 1 1-e 1-e 0+e],c3);plot([0 1 1 0 0],[0 0 1 1 0]);disp('Weights');
  "IW{1,1}(8,:)'" : Constant  Value=[-0.5655388403489804982626765195163898169994354248046875;-0.6331616038032603643870288578909821808338165283203125;-0.44882428912257221753634439664892852306365966796875;0.308823083232682815690850475220941007137298583984375;-0.276500535163689387108121309211128391325473785400390625;-0.31382172658632534467670893718604929745197296142578125;0.70661948398058738174398740738979540765285491943359375;-0.415865278039985242219955807740916498005390167236328125;-0.236564887738019036245162851628265343606472015380859375;-0.196415711695675010428630002934369258582592010498046875]
      mask Display: e = 0.06;c1 = [120 150 230]/255;c2 = ([120 150 230]+0)/383;c3 = ([120 150 230]+128)/383;patch([0 1 1 0],[0 0 1 1],c1);patch([0 1 1 1-e 1-e 0+e],[0 0 1 1-e 0+e 0+e],c2);patch([0 0 1 1-e 0+e 0+e],[0 1 1 1-e 1-e 0+e],c3);plot([0 1 1 0 0],[0 0 1 1 0]);disp('Weights');
  "IW{1,1}(9,:)'" : Constant  Value=[-0.5047369730512623053897414138191379606723785400390625;0.57787787424211967124421107655507512390613555908203125;-0.7925971254872414828440696510369889438152313232421875;0.234310215261569643185879385782754980027675628662109375;-0.53885470390463385825796649442054331302642822265625;-0.106781416498739012421737015756662003695964813232421875;0.523224110359839844619500581757165491580963134765625;0.3154159598341730319503994905971921980381011962890625;0.160680257492424427567812017514370381832122802734375;0.02605056733837439464362972785238525830209255218505859375]
      mask Display: e = 0.06;c1 = [120 150 230]/255;c2 = ([120 150 230]+0)/383;c3 = ([120 150 230]+128)/383;patch([0 1 1 0],[0 0 1 1],c1);patch([0 1 1 1-e 1-e 0+e],[0 0 1 1-e 0+e 0+e],c2);patch([0 0 1 1-e 0+e 0+e],[0 1 1 1-e 1-e 0+e],c3);plot([0 1 1 0 0],[0 0 1 1 0]);disp('Weights');
  Mux : Mux  Inputs=30
      mask Display: e = 0.06;c1 = [120 150 230]/255;c2 = ([120 150 230]+0)/383;c3 = ([120 150 230]+128)/383;patch([0 1 1 0],[0 0 1 1],c1);patch([0 1 1 1-e 1-e 0+e],[0 0 1 1-e 0+e 0+e],c2);patch([0 0 1 1-e 0+e 0+e],[0 1 1 1-e 1-e 0+e],c3);plot([0 1 1 0 0],[0 0 1 1 0]);disp('Mux');
  dotprod{1..30} (30 alike) : neural/Weight Functions/dotprod
  "iz{1,1}" : Outport
      mask Display: e = 0.06;c1 = [120 230 180]/255;c2 = ([120 230 180]+0)/(256+128);c3 = ([120 230 180]+128)/(256+128);patch([0 1 1 0],[0 0 1 1],c1);patch([0 1 1 1-e 1-e 0+e],[0 0 1 1-e 0+e 0+e],c2);patch([0 0 1 1-e 0+e 0+e],[0 1 1 1-e 1-e 0+e],c3);plot([0 1 1 0 0],[0 0 1 1 0]);
  wires:
  "IW{1,1}(1,:)'"/1 -> dotprod1/1
  "pd{1,1}"/1 -> dotprod1/2, dotprod2/2, dotprod3/2, dotprod4/2, dotprod5/2, dotprod6/2, dotprod7/2, dotprod8/2, dotprod9/2, dotprod10/2, dotprod11/2, dotprod12/2, dotprod13/2, dotprod14/2, dotprod15/2, dotprod16/2, dotprod17/2, dotprod18/2, dotprod19/2, dotprod20/2, dotprod21/2, dotprod22/2, dotprod23/2, dotprod24/2, dotprod25/2, dotprod26/2, dotprod27/2, dotprod28/2, dotprod29/2, dotprod30/2
  dotprod1/1 -> Mux/1
  "IW{1,1}(2,:)'"/1 -> dotprod2/1
  dotprod2/1 -> Mux/2
  "IW{1,1}(3,:)'"/1 -> dotprod3/1
  dotprod3/1 -> Mux/3
  "IW{1,1}(4,:)'"/1 -> dotprod4/1
  dotprod4/1 -> Mux/4
  "IW{1,1}(5,:)'"/1 -> dotprod5/1
  dotprod5/1 -> Mux/5
  "IW{1,1}(6,:)'"/1 -> dotprod6/1
  dotprod6/1 -> Mux/6
  "IW{1,1}(7,:)'"/1 -> dotprod7/1
  dotprod7/1 -> Mux/7
  "IW{1,1}(8,:)'"/1 -> dotprod8/1
  dotprod8/1 -> Mux/8
  "IW{1,1}(9,:)'"/1 -> dotprod9/1
  dotprod9/1 -> Mux/9
  "IW{1,1}(10,:)'"/1 -> dotprod10/1
  dotprod10/1 -> Mux/10
  "IW{1,1}(11,:)'"/1 -> dotprod11/1
  dotprod11/1 -> Mux/11
  "IW{1,1}(12,:)'"/1 -> dotprod12/1
  dotprod12/1 -> Mux/12
  "IW{1,1}(13,:)'"/1 -> dotprod13/1
  dotprod13/1 -> Mux/13
  "IW{1,1}(14,:)'"/1 -> dotprod14/1
  dotprod14/1 -> Mux/14
  "IW{1,1}(15,:)'"/1 -> dotprod15/1
  dotprod15/1 -> Mux/15
  "IW{1,1}(16,:)'"/1 -> dotprod16/1
  dotprod16/1 -> Mux/16
  "IW{1,1}(17,:)'"/1 -> dotprod17/1
  dotprod17/1 -> Mux/17
  "IW{1,1}(18,:)'"/1 -> dotprod18/1
  dotprod18/1 -> Mux/18
  "IW{1,1}(19,:)'"/1 -> dotprod19/1
  dotprod19/1 -> Mux/19
  "IW{1,1}(20,:)'"/1 -> dotprod20/1
  dotprod20/1 -> Mux/20
  "IW{1,1}(21,:)'"/1 -> dotprod21/1
  dotprod21/1 -> Mux/21
  "IW{1,1}(22,:)'"/1 -> dotprod22/1
  dotprod22/1 -> Mux/22
  "IW{1,1}(23,:)'"/1 -> dotprod23/1
  dotprod23/1 -> Mux/23
  "IW{1,1}(24,:)'"/1 -> dotprod24/1
  dotprod24/1 -> Mux/24
  "IW{1,1}(25,:)'"/1 -> dotprod25/1
  dotprod25/1 -> Mux/25
  "IW{1,1}(26,:)'"/1 -> dotprod26/1
  dotprod26/1 -> Mux/26
  "IW{1,1}(27,:)'"/1 -> dotprod27/1
  dotprod27/1 -> Mux/27
  "IW{1,1}(28,:)'"/1 -> dotprod28/1
  dotprod28/1 -> Mux/28
  "IW{1,1}(29,:)'"/1 -> dotprod29/1
  dotprod29/1 -> Mux/29
  "IW{1,1}(30,:)'"/1 -> dotprod30/1
  dotprod30/1 -> Mux/30
  Mux/1 -> "iz{1,1}"/1

== system mrefrobotarm_previous_y_previous_u_previous_ref_cover_test_2/Feed-Forward Neural Network1/Layer 2/Delays 1 ==
  "p{2}" : Inport  PortDimensions=30
      mask Display: e = 0.06;c1 = [120 230 180]/255;c2 = ([120 230 180]+0)/(256+128);c3 = ([120 230 180]+128)/(256+128);patch([0 1 1 0],[0 0 1 1],c1);patch([0 1 1 1-e 1-e 0+e],[0 0 1 1-e 0+e 0+e],c2);patch([0 0 1 1-e 0+e 0+e],[0 1 1 1-e 1-e 0+e],c3);plot([0 1 1 0 0],[0 0 1 1 0]);
  mux : Mux  Inputs=1
      mask Display: e = 0.06;c1 = [120 150 230]/255;c2 = ([120 150 230]+0)/383;c3 = ([120 150 230]+128)/383;patch([0 1 1 0],[0 0 1 1],c1);patch([0 1 1 1-e 1-e 0+e],[0 0 1 1-e 0+e 0+e],c2);patch([0 0 1 1-e 0+e 0+e],[0 1 1 1-e 1-e 0+e],c3);plot([0 1 1 0 0],[0 0 1 1 0]);disp('Mux')
  "pd{2,1}" : Outport
      mask Display: e = 0.06;c1 = [120 230 180]/255;c2 = ([120 230 180]+0)/(256+128);c3 = ([120 230 180]+128)/(256+128);patch([0 1 1 0],[0 0 1 1],c1);patch([0 1 1 1-e 1-e 0+e],[0 0 1 1-e 0+e 0+e],c2);patch([0 0 1 1-e 0+e 0+e],[0 1 1 1-e 1-e 0+e],c3);plot([0 1 1 0 0],[0 0 1 1 0]);
  wires:
  "p{2}"/1 -> mux/1
  mux/1 -> "pd{2,1}"/1
